simulink model "Adelantamientov3"  (R2019b)
settings: Solver=FixedStepDiscrete  StartTime=0.0  StopTime=15  RelTol=1e-3
model workspace (MAT data in the model file):
  firstWarning = 1
  originalScenarioChecksum = '158070AB835E3E5B039703679FDCB6FF'
values from neighbouring files (symbols this model uses):
  fault_d = 200    [initialize.m]
  P_ego_init = -200    [initialize.m]
  t_gap = 1.5    [initialize.m]
  V_ego_init = 90/3.6    (= 25)    [initialize.m]
undefined symbols (not defined in the file or in its folder): DiscIntNeverNeededParam, driving
libraries: drivingscenarioandsensors x3, drivinglib x2, mpcadaslib x1
settings Model: Creator=Sun Tzu  LastModifiedBy=Sun Tzu

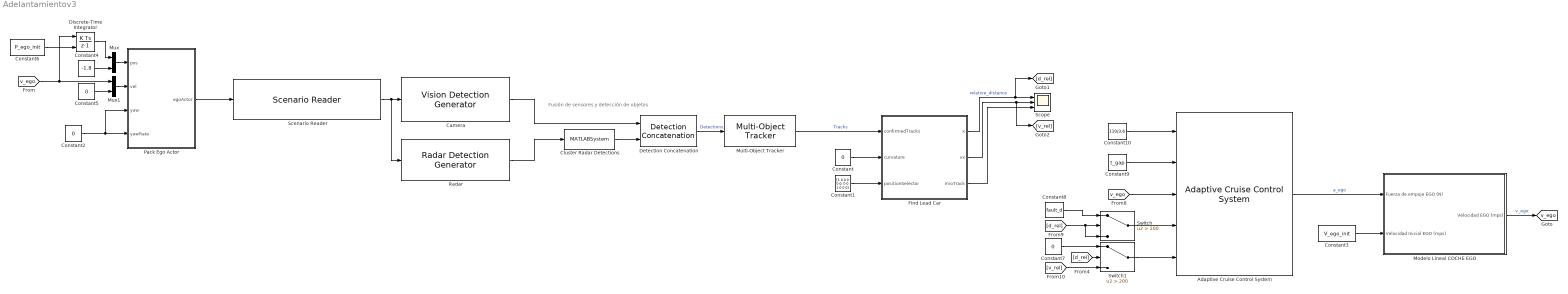
== system Adelantamientov3 ==
  note: Fusión de sensores y detección de objetos
  Adaptive Cruise Control System : mpcadaslib/Adaptive Cruise Control System  EgoModel=tf(0.05,[81.1,1])  InitialEgoVelocity=110/3.6  DefaultSpacing=10  MaxVelocity=120/3.6  MinAcceleration=-3000  amin_ext=off  MaxAcceleration=2000  amax_ext=off  Ts=0.1  PredictionHorizon=30  ControllerBehavior=0.700  suboptimal=off  maxiter=10  datatypeopt=double  optmode=off  trackmode=off
      settings: SourceProductName=Model Predictive Control Toolbox
  Camera : drivingscenarioandsensors/Vision Detection Generator  SensorIndex=1  DetectorOutput=Objects only  UpdateInterval=0.1  LaneUpdateInterval=0.1  SensorLocation=[1.9 0]  Height=1.1  Yaw=0  Pitch=1  Roll=0  BusNameSource=Auto  BusName=BusObjectDetections  BusName2Source=Auto  BusName2=BusLaneDetections  MaxNumDetectionsSource=Property  MaxNumDetections=50  MaxNumLanesSource=Property  MaxNumLanes=30  DetectionCoordinates=Ego Cartesian  SimulateUsing=Interpreted execution  MaxRange=100  BoundingBoxAccuracy=5  ProcessNoiseIntensity=5  MaxSpeed=50  MaxAllowedOcclusion=0.5  MinObjectImageSize=[15 15]  DetectionProbability=0.9  FalsePositivesPerImage=0.1  MinLaneImageSize=[20 3]  LaneBoundaryAccuracy=3  HasNoise=on  InitialSeedSource=Repeatable  InitialSeed=0  UsedSeed=0  ActorProfilesSource=MATLAB expression  ActorProfilesParameters=driving.internal.ActorProfilesParameters  ActorProfilesExpression=[struct('ActorID',1,'ClassID',6,'Length',4.7,'Width',1.8,'Height',1.4,'OriginOffset',[-1.35 0 0],'RCSPattern',[10 10;10 10],'RCSAzimuthAngles',[-180 180],'RCSElevationAngles',[-90 90]); struct('ActorID',2,'ClassID',2,'Length',8.2,'Width',2.5,'Height',3.5,'OriginOffset',[-3.1 0 0],'RCSPattern',[10 10;10 10],'RCSAzimuthAngles',[-180 180],'RCSElevationAngles',[-90 90]); struct('ActorID',3,'ClassID',2,'Length',8.2,'Width',2.5,'Height',3.5,'OriginOffset',[-3.1 0 0],'RCSPattern',[10 10;10 10],'RCSAzimuthAngles',[-180 180],'RCSElevationAngles',[-90 90]); struct('ActorID',4,'ClassID',1,'Length',4.7,'Width',1.8,'Height',1.4,'OriginOffset',[-1.35 0 0],'RCSPattern',[10 10;10 10],'RCSAzimuthAngles',[-180 180],'RCSElevationAngles',[-90 90])]  Intrinsics=driving.internal.cameraIntrinsics('FocalLength',[1814.81018227767 1814.81018227767],'PrincipalPoint',[320 240],'ImageSize',[480 640],'RadialDistortion',[0 0],'TangentialDistortion',[0 0],'Skew',0)
      settings: SourceProductName=Automated Driving Toolbox
  Cluster Radar Detections : MATLABSystem  System=helperClusterDetections  ClusterSize=5  BusNameSource=Auto  BusName=BusClusterDetections  SimulateUsing=Interpreted execution
      mask Type: helperClusterDetections
      mask Display:
      | disp(['Detection' char(10) 'Clustering']);
      | port_label('input',1,'In');
      | port_label('output',1,'Out');
  Constant{,2,5,7} (4 alike) : Constant  Value=0
  Constant1 : Constant  Value=[1 0 0 0 0 0; 0 0 1 0 0 0]
  Constant10 : Constant  Value=110/3.6
  Constant3 : Constant  Value=V_ego_init
  Constant4 : Constant  Value=-1.8
  Constant6 : Constant  Value=P_ego_init
  Constant8 : Constant  Value=fault_d
  Constant9 : Constant  Value=t_gap
  Detection Concatenation : drivinglib/Detection Concatenation  NumInputs=2  BusNameSource=Auto  BusName=BusDetectionConcatenation1  SimulateUsing=Interpreted execution
      settings: SourceProductName=Automated Driving Toolbox  SourceProductBaseCode=DR
  Discrete-Time Integrator : DiscreteIntegrator  InitialConditionSource=external  InitialCondition=5  SampleTime=-1  ICPrevOutput=DiscIntNeverNeededParam  ICPrevScaledInput=DiscIntNeverNeededParam
  Find Lead Car : MATLAB Function  TreatAsAtomicUnit=on
  Modelo Lineal COCHE EGO : Subsystem
  Multi-Object Tracker : drivinglib/Multi-Object Tracker  FilterInitializationFcn=helperInitSimulinkDemoFilter  AssignmentThreshold=50  ConfirmationParameters=[ 2, 3 ]  NumCoastingUpdates=5  MaxNumTracks=20  MaxNumSensors=8  TimeInputSource=Auto  HasCostMatrixInput=off  BusNameSource=Auto  BusName=BusMultiObjectTracker1  TentativeTracksOutputPort=off  AllTracksOutputPort=off  SimulateUsing=Interpreted execution
      settings: SourceProductName=Automated Driving Toolbox  SourceProductBaseCode=DR
  Mux : Mux  Inputs=2
  Mux1 : Mux  Inputs=2
  Pack Ego Actor : MATLAB Function  TreatAsAtomicUnit=on
  Radar : drivingscenarioandsensors/Radar Detection Generator  SensorIndex=2  UpdateInterval=0.1  SensorLocation=[3.7 0]  Height=0.2  Yaw=0  Pitch=0  Roll=0  BusNameSource=Auto  BusName=BusRadarDetectionGenerator  MaxNumDetectionsSource=Property  MaxNumDetections=50  DetectionCoordinates=Ego Cartesian  SimulateUsing=Interpreted execution  AzimuthResolution=4  ElevationResolution=10  RangeResolution=2.5  RangeRateResolution=0.5  AzimuthBiasFraction=0.1  ElevationBiasFraction=0.1  RangeBiasFraction=0.05  RangeRateBiasFraction=0.05  FieldOfView=[10 5]  MaxRange=200  RangeRateLimits=[-100 100]  DetectionProbability=0.9  FalseAlarmRate=1e-06  ReferenceRange=150  ReferenceRCS=0  HasElevation=off  HasRangeRate=on  HasNoise=on  HasFalseAlarms=on  HasOcclusion=on  InitialSeedSource=Repeatable  InitialSeed=0  UsedSeed=0  ActorProfilesSource=MATLAB expression  ActorProfilesParameters=driving.internal.ActorProfilesRadarParameters  ActorProfilesExpression=[struct('ActorID',1,'ClassID',6,'Length',4.7,'Width',1.8,'Height',1.4,'OriginOffset',[-1.35 0 0],'RCSPattern',[10 10;10 10],'RCSAzimuthAngles',[-180 180],'RCSElevationAngles',[-90 90]); struct('ActorID',2,'ClassID',2,'Length',8.2,'Width',2.5,'Height',3.5,'OriginOffset',[-3.1 0 0],'RCSPattern',[10 10;10 10],'RCSAzimuthAngles',[-180 180],'RCSElevationAngles',[-90 90]); struct('ActorID',3,'ClassID',2,'Length',8.2,'Width',2.5,'Height',3.5,'OriginOffset',[-3.1 0 0],'RCSPattern',[10 10;10 10],'RCSAzimuthAngles',[-180 180],'RCSElevationAngles',[-90 90]); struct('ActorID',4,'ClassID',1,'Length',4.7,'Width',1.8,'Height',1.4,'OriginOffset',[-1.35 0 0],'RCSPattern',[10 10;10 10],'RCSAzimuthAngles',[-180 180],'RCSElevationAngles',[-90 90])]
      settings: SourceProductName=Automated Driving Toolbox  SourceProductBaseCode=DR
  Scenario Reader : drivingscenarioandsensors/Scenario Reader  ScenarioSource=From file  ScenarioFileName=D:\Sun Tzu\Documents\MIERA\CdV\ControlVehiculosMPC-master\Escenario_Sensores\EscenarioAdelantamiento.mat  ScenarioVariableName=scenario  OutputCoordinateSystem=Vehicle coordinates  EgoVehicleSource=Input port  EgoVehicleActorID=1  SampleTime=0.1  LaneBoundaryOutput=None  LaneBoundaryDistance=0:0.5:9.5  LaneBoundaryLocation=Center of lane markings  BusNameSource=Auto  BusName=BusActorsActors  BusName2Source=Auto  BusName2=BusLaneBoundaries  SimulateUsing=Interpreted execution
      settings: SourceProductName=Automated Driving Toolbox
  Scope : Scope  NumInputPorts=3
  Switch : Switch  Criteria=u2 > Threshold  Threshold=200
  Switch1 : Switch  Criteria=u2 > Threshold  Threshold=200
  tag scope: v_ego=global
  wires:
  Scenario Reader/1 -> Camera/1, Radar/1
  Find Lead Car/2(vx) -> [v_rel], Scope/2
  Multi-Object Tracker/1 -> Find Lead Car/1(confirmedTracks)  "Tracks"
  Cluster Radar Detections/1 -> Detection Concatenation/2
  Detection Concatenation/1 -> Multi-Object Tracker/1  "Detections"
  Find Lead Car/3(mioTrack) -> Scope/3
  Radar/1 -> Cluster Radar Detections/1
  Constant/1 -> Find Lead Car/2(curvature)
  Camera/1 -> Detection Concatenation/1
  Constant1/1 -> Find Lead Car/3(positionSelector)
  Find Lead Car/1(x) -> [d_rel], Scope/1  "relative_distance"
  Pack Ego Actor/1(egoActor) -> Scenario Reader/1
  Constant2/1 -> Pack Ego Actor/3(yaw), Pack Ego Actor/4(yawRate)
  [v_ego] -> Discrete-Time Integrator/1, Mux1/1
  Discrete-Time Integrator/1 -> Mux/1
  Mux/1 -> Pack Ego Actor/1(pos)
  Constant4/1 -> Mux/2
  Mux1/1 -> Pack Ego Actor/2(vel)
  Constant5/1 -> Mux1/2
  Constant8/1 -> Switch/1
  Switch/1 -> Adaptive Cruise Control System/4
  [d_rel] -> Switch1/2
  Constant7/1 -> Switch1/1
  [v_rel] -> Switch1/3
  [d_rel] -> Switch/3, Switch/2
  Switch1/1 -> Adaptive Cruise Control System/5
  [v_ego] -> Adaptive Cruise Control System/3
  Adaptive Cruise Control System/1 -> Modelo Lineal COCHE EGO/1(Fuerza de empuje EGO (N))  "a_ego"
  Constant10/1 -> Adaptive Cruise Control System/1
  Constant9/1 -> Adaptive Cruise Control System/2
  Modelo Lineal COCHE EGO/1(Velocidad EGO (mps)) -> [v_ego]  "v_ego"
  Constant3/1 -> Modelo Lineal COCHE EGO/2(Velocidad Inicial EGO (mps))
  Constant6/1 -> Discrete-Time Integrator/2

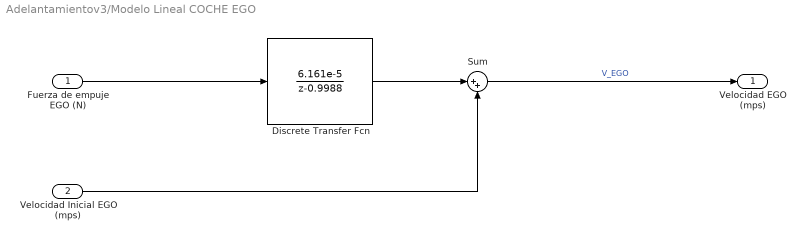
== system Adelantamientov3/Modelo Lineal COCHE EGO ==
  Fuerza de empuje EGO (N) : Inport
  Velocidad Inicial EGO (mps) : Inport  Port=2
  Discrete Transfer Fcn : DiscreteTransferFcn  Numerator=[6.161e-5]  Denominator=[1 -0.9988]  SampleTime=0.1
  Sum : Sum  Inputs=|++
  Velocidad EGO (mps) : Outport  VectorParamsAs1DForOutWhenUnconnected=off
  wires:
  Discrete Transfer Fcn/1 -> Sum/1
  Sum/1 -> Velocidad EGO (mps)/1  "V_EGO"
  Velocidad Inicial EGO (mps)/1 -> Sum/2
  Fuerza de empuje EGO (N)/1 -> Discrete Transfer Fcn/1

== matlab function Adelantamientov3/Find Lead Car ==
  data: confirmedTracks input; x output double size=[1 1]; vx output size=[1 1]; curvature input; mioTrack output; positionSelector input
function [x,vx,mioTrack] = findLeadCar(confirmedTracks, curvature, positionSelector)
% This function finds the lead car: a car in front of the ego car that
% satisfies all the criteria below:
% * Within the ego car's lane.
% * In front of the ego car.
% * Closest to the ego car.

% Important notes:
% 1. If you change state definition, change the following:
%       State = [x;vx;y;vy;z;vz] (3D constant velocity)
numStates = 6;

% 2. The lane is defined using a parabolic model, where y=ax^2+bx+c. a is
%    equal to half the road curvature, b=0, and c is the offset of the lane
%    boundaries relative to the ego car. Overall lane width is assumed to
%    be 3.6m, typical highway lane width.
laneWidth = 3.6;

% 3. The ego car is assumed to be traveling in the middle of its lane, with
%    1.8m on each side of it. So, c=+1.8m for the left lane boundary and
%    -1.8m for the right lane boundary.
halfLaneWidth = laneWidth/2;

% Initialize outputs and parameters
maxX = cast(1000, 'like', confirmedTracks.Tracks(1).State);  % Far enough forward so that no track is expected to exceed this distance
trackID = 0;

for i = 1:confirmedTracks.NumTracks
    position = positionSelector * confirmedTracks.Tracks(i).State;
    x = position(1); % Longitudinal position of the track relative to ego
    y = position(2); % Lateral position of the track relative to ego
    
    if x < maxX && x > 0 % No point checking otherwise
        yleftLane  = polyval([curvature/2, 0,  halfLaneWidth],x); % Half a lane to the left
        yrightLane = polyval([curvature/2, 0, -halfLaneWidth],x); % Half a lane to the right
        
        % Find a new lead car
        if (yrightLane <= y) && (y <= yleftLane)
            maxX = x;
            trackID = i;
        end
    end
end

if trackID>0
    mioState = confirmedTracks.Tracks(trackID).State;
else
    mioState = inf(numStates,1,'like',confirmedTracks.Tracks(1).State);
end

% Output:
x = mioState(1);    % Longitudinal position of the lead car
vx = mioState(2);   % Longitudinal velocity of the lead car
mioTrack = trackID; % Index of the most important track

== matlab function Adelantamientov3/Pack Ego Actor ==
  data: pos input; egoActor output Bus: BusActors1Actors size=1; vel input; yaw input; yawRate input
function egoActor = packEgo(pos,vel,yaw,yawRate)
% Pack ego information into a single ego actor bus
%
% Imoprtant note:
% Output is a bus of type BusActorsActors. This is the same bus used by the
% Scenario Reader to output an individual actor. If you change the
% output bus name of Scenario Reader, change the output bus name here
% as well by clicking on 'Edit Data' in the menu above.

egoActor = struct(...
    'ActorID',1,...
    'Position', [pos(1) pos(2) 0], ...
    'Velocity', [vel(1) vel(2) 0], ...
    'Roll', 0, ...
    'Pitch', 0, ...
    'Yaw', yaw, ...
    'AngularVelocity', [0 0 yawRate]);
